simulink model "test_controller"  (R2020a)
settings: Solver=ode1  StartTime=0.0  StopTime=100  FixedStep=0.01  RelTol=1e-3
InitFcn:
  | Initialization;
values from neighbouring files (symbols this model uses):
  ics = JsonLoad('ics.json')    [Initialization.m]
  params = JsonLoad('params.json')    [Initialization.m]
undefined symbols (not defined in the file or in its folder): sim_, U_initial
libraries: sharedtransform x2, dspinverses x2, simulink x2, dspmtrx3 x1, sharedutil x1
(part 1 of 2)
settings Model: NumberOfSteps=100  Creator=arthus  LastModifiedBy=hs293go
settings DataIOCC: ReturnWorkspaceOutputs=off
settings DebuggingCC: ArithmeticOperatorsInVariantConditions=warning
settings SFSimCC: SimUseLocalCustomCode=off  CustomCodeUndefinedFunction=UseInterfaceOnly
settings RTWCC: RTWUseLocalCustomCode=off
settings CodeAppCC: StateflowObjectComments=on

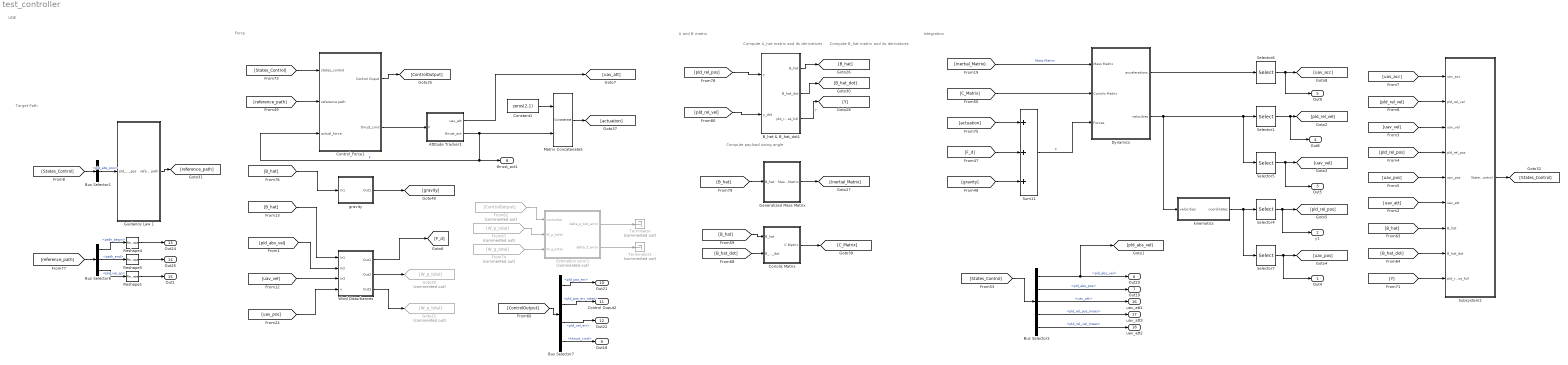
== system test_controller ==
  note: Compute B_hat matrix and its derivatives
  note: Force
  note: A and B matrix
  note: Target Path
  note: Compute A_hat matrix and its derivatives
  note: Integration
  note: Compute payload swing angle
  note: UDE
  Attitude Tracker1 : Subsystem
  B_hat & B_hat_dot1 : Subsystem
  Bus Selector1 : BusSelector  OutputSignals=pld_abs_pos
  Bus Selector2 : BusSelector  OutputSignals=pld_abs_vel,pld_abs_pos,uav_att,pld_rel_pos_meas,pld_rel_vel_meas
  Bus Selector6 : BusSelector  OutputSignals=path_begin,path_end,pld_vel_sp
  Bus Selector7 : BusSelector  OutputSignals=pld_pos_err,pld_pos_err_rates,pld_vel_err,thrust_cmd
  Constant1 : Constant  Value=zeros(2,1)
  Control_Force1 : Subsystem
  Coriolis Matrix : Subsystem
  Dynamics : Subsystem
  Estimation error1 : Subsystem  Commented=on
  From62 : From  Commented=on  GotoTag=ControlOutput
  From67 : From  Commented=on  GotoTag=W_p_total
  From74 : From  Commented=on  GotoTag=W_q_total
  Generalized Mass Matrix : Subsystem
  Goto20 : Goto  Commented=on  GotoTag=W_p_total
  Goto22 : Goto  Commented=on  GotoTag=W_q_total
  Guidance Law 1 : Subsystem
  Matrix Concatenate5 : Concatenate  Mode=Multidimensional array
  Reshape1 : Reshape  OutputDimensionality=Column vector (2-D)
  Reshape4 : Reshape  OutputDimensionality=Column vector (2-D)
  Reshape5 : Reshape  OutputDimensionality=Column vector (2-D)
  Selector1 : Selector  InputPortWidth=5  IndexOptions=Index vector (dialog)  Indices=[1 2]  OutputSizes=1
  Selector4 : Selector  InputPortWidth=5  IndexOptions=Index vector (dialog)  Indices=[1 2]  OutputSizes=1
  Selector5 : Selector  InputPortWidth=5  IndexOptions=Index vector (dialog)  Indices=[3 4 5]  OutputSizes=1
  Selector6 : Selector  InputPortWidth=5  IndexOptions=Index vector (dialog)  Indices=[3 4 5]  OutputSizes=1
  Selector7 : Selector  InputPortWidth=5  IndexOptions=Index vector (dialog)  Indices=[3 4 5]  OutputSizes=1
  Subsystem2 : Subsystem
  Sum11 : Sum  Inputs=+++
  Terminator : Terminator  Commented=on
  Terminator2 : Terminator  Commented=on
  Wind Disturbances : Subsystem
  gravity : Subsystem
  kinematics : Subsystem
  Out4 : Outport  SignalName=uav_pos
  y1 : Outport  Port=2  SignalName=pld_rel_pos
  Out5 : Outport  Port=3  SignalName=uav_vel
  Out8 : Outport  Port=4  SignalName=pld_rel_vel
  Out9 : Outport  Port=5  SignalName=uav_acc
  Out20 : Outport  Port=6  SignalName=pld_abs_vel
  Out19 : Outport  Port=7  SignalName=pld_abs_pos
  thrust_act1 : Outport  Port=8  SignalName=thrust_act  VectorParamsAs1DForOutWhenUnconnected=off
  Out18 : Outport  Port=9  SignalName=thrust_cmd
  Out21 : Outport  Port=10  SignalName=pld_pos_err
  Control Ouput2 : Outport  Port=11  SignalName=pld_pos_err_rates
  Out22 : Outport  Port=12  SignalName=pld_vel_err
  Out24 : Outport  Port=13  SignalName=path_begin
  Out25 : Outport  Port=14  SignalName=path_end
  Out1 : Outport  Port=15  SignalName=pld_vel_sp
  uav_att1 : Outport  Port=16  SignalName=uav_att  VectorParamsAs1DForOutWhenUnconnected=off
  uav_att3 : Outport  Port=17  SignalName=pld_rel_pos_meas  VectorParamsAs1DForOutWhenUnconnected=off
  uav_att2 : Outport  Port=18  SignalName=pld_rel_vel_meas  VectorParamsAs1DForOutWhenUnconnected=off
  wires:
  Control_Force1/1(Control Ouput) -> [ControlOutput]
  Reshape5/1 -> Out25/1
  Constant1/1 -> Matrix Concatenate5/1
  Subsystem2/1(States_Control) -> [States_Control]
  B_hat & B_hat_dot1/2(B_hat_dot) -> [B_hat_dot]
  [B_hat] -> gravity/1(In1)
  Bus Selector6/1 -> Reshape4/1  "<path_begin>"
  Selector5/1 -> [uav_vel], Out5/1
  [Inertial_Matrix] -> Dynamics/1(Mass Matrix)  "Mass Matrix"
  Attitude Tracker1/2(thrust_act) -> Control_Force1/3(actual_force), thrust_act1/1, Matrix Concatenate5/2  "F"
  [reference_path] -> Control_Force1/2(reference path)
  [gravity] -> Sum11/3
  [B_hat] -> Generalized Mass Matrix/1(B_hat)
  Selector7/1 -> [uav_pos], Out4/1
  Bus Selector7/3 -> Out22/1  "<pld_vel_err>"
  Bus Selector2/1 -> [pld_abs_vel], Out20/1  "<pld_abs_vel>"
  From67/1 -> Estimation error1/2(W_p_total)
  Coriolis Matrix/1(C Matrix) -> [C_Matrix]
  Bus Selector2/2 -> Out19/1  "<pld_abs_pos>"
  Dynamics/2(velocities) -> kinematics/1(velocities), Selector5/1, Selector1/1
  [F_d] -> Sum11/2
  [B_hat] -> Subsystem2/7(B_hat)
  Generalized Mass Matrix/1(Mass Matrix) -> [Inertial_Matrix]
  [B_hat_dot] -> Subsystem2/8(B_hat_dot)
  Selector6/1 -> [uav_acc], Out9/1
  Bus Selector6/2 -> Reshape5/1  "<path_end>"
  Sum11/1 -> Dynamics/3(Forces)  "F"
  [Y] -> Subsystem2/9(pld_rel_pos_full)
  Control_Force1/2(thrust_cmd) -> Attitude Tracker1/1(F)
  Selector1/1 -> Out8/1, [pld_rel_vel]
  Matrix Concatenate5/1 -> [actuation]
  [actuation] -> Sum11/1
  B_hat & B_hat_dot1/3(pld_rel_pos_full) -> [Y]  "Y"
  [States_Control] -> Bus Selector2/1
  [ControlOutput] -> Bus Selector7/1
  [pld_rel_pos] -> B_hat & B_hat_dot1/1(y)
  Bus Selector7/2 -> Control Ouput2/1  "<pld_pos_err_rates>"
  [reference_path] -> Bus Selector6/1
  Guidance Law 1/1(reference path) -> [reference_path]
  [States_Control] -> Control_Force1/1(states_control)
  [C_Matrix] -> Dynamics/2(Coriolis Matrix)
  Selector4/1 -> [pld_rel_pos], y1/1
  kinematics/1(coordinates) -> Selector7/1, Selector4/1
  B_hat & B_hat_dot1/1(B_hat) -> [B_hat]
  [pld_rel_vel] -> B_hat & B_hat_dot1/2(y_dot)
  Dynamics/1(accelerations) -> Selector6/1
  Bus Selector7/1 -> Out21/1  "<pld_pos_err>"
  [B_hat] -> Coriolis Matrix/1(B_hat)
  Reshape4/1 -> Out24/1
  [B_hat_dot] -> Coriolis Matrix/2(B_hat_dot)
  Attitude Tracker1/1(uav_att) -> [uav_att]
  gravity/1(Out1) -> [gravity]
  From62/1 -> Estimation error1/1(controller)
  From74/1 -> Estimation error1/3(W_q_total)
  [B_hat] -> Wind Disturbances/1(In1)
  [uav_vel] -> Wind Disturbances/3(In3)
  [uav_pos] -> Wind Disturbances/4(x)
  Wind Disturbances/1(Out1) -> [F_d]
  Wind Disturbances/2(Out2) -> Goto20/1
  Wind Disturbances/3(Out3) -> Goto22/1
  Estimation error1/1(delta_p_bot_error) -> Terminator/1
  Estimation error1/2(delta_T_error) -> Terminator2/1
  [uav_att] -> Subsystem2/6(uav_att)
  Bus Selector2/3 -> uav_att1/1  "<uav_att>"
  [uav_vel] -> Subsystem2/3(uav_vel)
  [pld_rel_pos] -> Subsystem2/4(pld_rel_pos)
  [uav_pos] -> Subsystem2/5(uav_pos)
  [pld_rel_vel] -> Subsystem2/2(pld_rel_vel)
  [uav_acc] -> Subsystem2/1(uav_acc)
  [pld_abs_vel] -> Wind Disturbances/2(In2)
  Bus Selector2/5 -> uav_att2/1  "<pld_rel_vel_meas>"
  Bus Selector2/4 -> uav_att3/1  "<pld_rel_pos_meas>"
  Bus Selector7/4 -> Out18/1  "<thrust_cmd>"
  [States_Control] -> Bus Selector1/1
  Bus Selector1/1 -> Guidance Law 1/1(pld_abs_pos)  "<pld_abs_pos>"
  Reshape1/1 -> Out1/1
  Bus Selector6/3 -> Reshape1/1  "<pld_vel_sp>"

== system test_controller/Attitude Tracker1 ==
  F : Inport
  Attitude Dynamics : Subsystem
  Attitude Tracker : Subsystem
  Atttitude Extraction : Subsystem
  Constant : Constant  Value=[0 0 1]'  VectorParams1D=off
  Divide : Product  Inputs=*/
  Dot Product : DotProduct  InputSameDT=on  OutDataTypeStr=Inherit: Inherit via internal rule
  Product : Product  Multiplication=Matrix(*)
  Product1 : Product
  Sqrt : Sqrt  SaturateOnIntegerOverflow=on
  Terminator : Terminator
  Terminator1 : Terminator
  uav_att : Outport
  thrust_act : Outport  Port=2  VectorParamsAs1DForOutWhenUnconnected=off
  wires:
  F/1 -> Dot Product/2, Dot Product/1, Divide/1
  Constant/1 -> Product/2
  Product/1 -> Product1/2  "n_z"
  Product1/1 -> thrust_act/1
  Sqrt/1 -> Product1/1, Divide/2
  Dot Product/1 -> Sqrt/1
  Atttitude Extraction/1(R_d) -> Attitude Tracker/1(R_d)
  Atttitude Extraction/2(omega_d) -> Attitude Tracker/2(omega_d)
  Atttitude Extraction/3(omega_d_dot) -> Attitude Tracker/3(omega_d_dot)
  Divide/1 -> Atttitude Extraction/1(n_d)  "n1"
  Attitude Dynamics/4(omega_b) -> Attitude Tracker/5(omega)
  Attitude Dynamics/3(Euler) -> Terminator1/1  "Euler"
  Attitude Dynamics/2(RBI) -> Terminator/1
  Attitude Tracker/1(Torque_in_body_frame) -> Attitude Dynamics/1(MB)  "Mq_b"
  Attitude Dynamics/1(RIB) -> uav_att/1, Attitude Tracker/4(R), Product/1  "IRB"

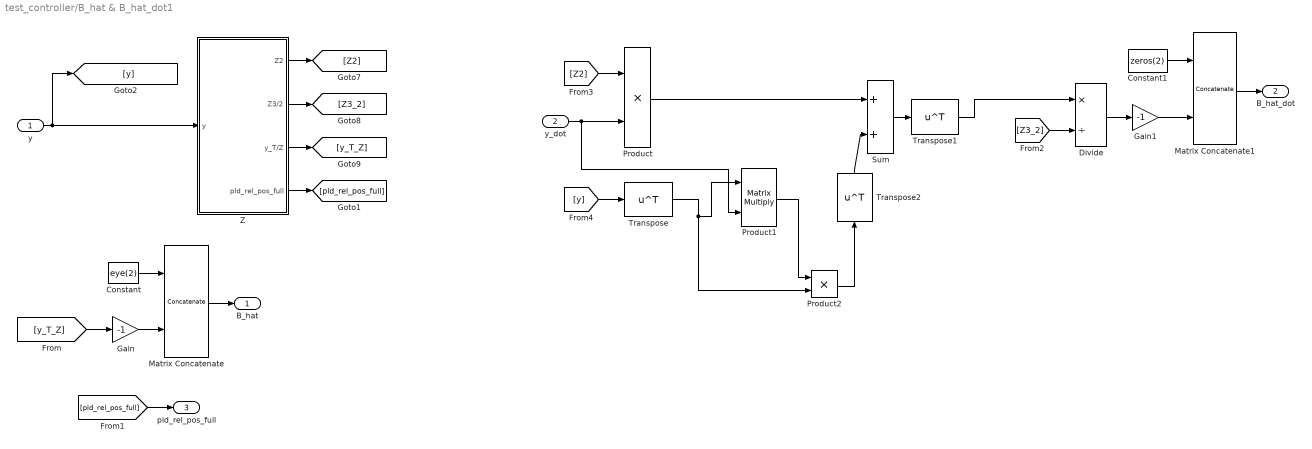
== system test_controller/B_hat & B_hat_dot1 ==
  y : Inport
  y_dot : Inport  Port=2
  Constant : Constant  Value=eye(2)
  Constant1 : Constant  Value=zeros(2)
  Divide : Product  Inputs=*/
  Gain : Gain  Gain=-1
  Gain1 : Gain  Gain=-1
  Matrix Concatenate : Concatenate  Mode=Multidimensional array
  Matrix Concatenate1 : Concatenate  Mode=Multidimensional array
  Product : Product  RndMeth=Zero
  Product1 : Product  Multiplication=Matrix(*)  RndMeth=Zero
  Product2 : Product  RndMeth=Zero
  Sum : Sum
  Transpose : Math  Operator=transpose  SignedPower=on  SaturateOnIntegerOverflow=on
  Transpose1 : Math  Operator=transpose  SignedPower=on  SaturateOnIntegerOverflow=on
  Transpose2 : Math  Operator=transpose  SignedPower=on  SaturateOnIntegerOverflow=on
  Z : Subsystem
  B_hat : Outport  VectorParamsAs1DForOutWhenUnconnected=off
  B_hat_dot : Outport  Port=2  VectorParamsAs1DForOutWhenUnconnected=off
  pld_rel_pos_full : Outport  Port=3  VectorParamsAs1DForOutWhenUnconnected=off
  wires:
  y_dot/1 -> Product/2, Product1/2
  y/1 -> Z/1(y), [y]
  Matrix Concatenate/1 -> B_hat/1
  Matrix Concatenate1/1 -> B_hat_dot/1
  Z/1(Z2) -> [Z2]
  Z/2(Z3/2) -> [Z3_2]
  Z/3(y_T/Z) -> [y_T_Z]
  [y_T_Z] -> Gain/1
  Constant/1 -> Matrix Concatenate/1
  Gain/1 -> Matrix Concatenate/2
  Z/4(pld_rel_pos_full) -> [pld_rel_pos_full]
  [pld_rel_pos_full] -> pld_rel_pos_full/1
  Constant1/1 -> Matrix Concatenate1/1
  [Z3_2] -> Divide/2
  Sum/1 -> Transpose1/1
  [Z2] -> Product/1
  [y] -> Transpose/1
  Transpose/1 -> Product1/1, Product2/2
  Product1/1 -> Product2/1
  Divide/1 -> Gain1/1
  Gain1/1 -> Matrix Concatenate1/2
  Product2/1 -> Transpose2/1
  Product/1 -> Sum/1
  Transpose1/1 -> Divide/1
  Transpose2/1 -> Sum/2

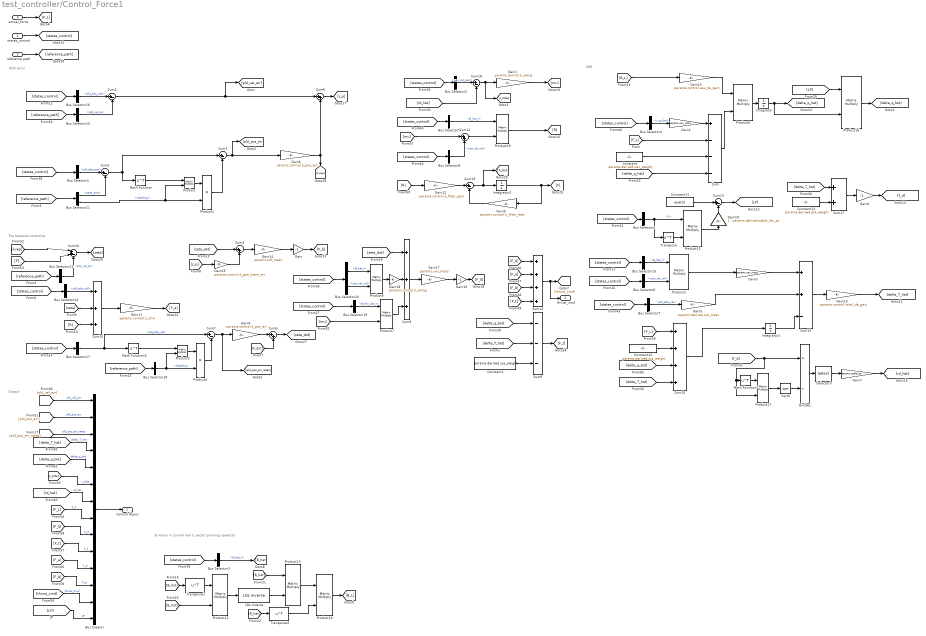
== system test_controller/Control_Force1 ==
  note: Output
  note: Path error
  note: The baseline controller
  note: B matrix in control law (L vector pointing upwards)
  note: UDE
  states_control : Inport
  reference path : Inport  Port=2
  actual_force : Inport  Port=3
  Bus Creator : BusCreator  Inputs=14
  Bus Selector1 : BusSelector  OutputSignals=pld_abs_pos
  Bus Selector10 : BusSelector  OutputSignals=pld_vel_sp
  Bus Selector11 : BusSelector  OutputSignals=path_end,heading
  Bus Selector13 : BusSelector  OutputSignals=pld_vel_sp
  Bus Selector{7,14,16..17} (4 alike) : BusSelector  OutputSignals=pld_abs_vel
  Bus Selector15 : BusSelector  OutputSignals=B_hat_l
  Bus Selector18 : BusSelector  OutputSignals=heading
  Bus Selector19 : BusSelector  OutputSignals=B_hat_dot_l
  Bus Selector2 : BusSelector  OutputSignals=uav_rel_pos
  Bus Selector20 : BusSelector  OutputSignals=B_hat_l,uav_rel_vel
  Bus Selector3 : BusSelector  OutputSignals=B_hat_l
  Bus Selector4 : BusSelector  OutputSignals=v_q_dot
  Bus Selector5 : BusSelector  OutputSignals=L
  Bus Selector6 : BusSelector  OutputSignals=uav_rel_vel
  Bus Selector8 : BusSelector  OutputSignals=uav_rel_vel
  Bus Selector9 : BusSelector  OutputSignals=B_hat_l
  Constant : Constant  Value=params.derived.uav_weight
  Constant1 : Constant  Value=params.derived.sys_weight
  Constant11 : Constant  Value=eye(3)
  Constant12 : Constant  Value=params.derived.sys_weight
  Constant13 : Constant  Value=params.derived.pld_weight
  Divide1 : Product  Inputs=*/
  Gain : Gain  Gain=-1
  Gain1 : Gain  Gain=params.control.k_swing
  Gain10 : Gain  Gain=params.control.uav_de_gain
  Gain11 : Gain  Gain=-params.control.k_trim
  Gain12 : Gain  Gain=params.control.k_filter_gain
  Gain13 : Gain  Gain=params.control.total_de_gain
  Gain14 : Gain  Gain=params.pld_mass
  Gain15 : Gain  Gain=params.control.k_gen_trans_err
  Gain16 : Gain  Gain=-1
  Gain17 : Gain  Gain=params.uav_mass
  Gain18 : Gain  Gain=params.control.k_swing
  Gain19 : Gain  Gain=1 / params.derived.cable_len_sq
  Gain2 : Gain  Gain=params.uav_mass
  Gain3 : Gain  Gain=params.uav_mass
  Gain4 : Gain  Gain=params.control.k_pos_err
  Gain5 : Gain  Gain=params.derived.sys_mass
  Gain6 : Gain  Gain=-1
  Gain7 : Gain  Gain=params.cable_len
  Gain8 : Gain  Gain=params.control.k_pos_err
  Gain9 : Gain  Gain=params.control.k_filter_leak
  Integrator : Integrator
  Integrator1 : Integrator
  Integrator2 : Integrator
  LDL Inverse : dspinverses/LDL Inverse  errmode=Error
      settings: SourceProductBaseCode=DS
  Math Function : Math  Operator=transpose  SignedPower=on  SaturateOnIntegerOverflow=on
  Math Function3 : Math  Operator=transpose  SignedPower=on  SaturateOnIntegerOverflow=on
  Math Function4 : Math  Operator=transpose  SignedPower=on  SaturateOnIntegerOverflow=on
  Product{,2..3,7..9,12..17,19} (13 alike) : Product  Multiplication=Matrix(*)
  Product1 : Product
  Product4 : Product
  Selector3 : Selector  InputPortWidth=3  IndexOptions=Index vector (dialog)  Indices=[1 2]  OutputSizes=1
  Sqrt6 : Sqrt  SaturateOnIntegerOverflow=on
  Sum : Sum  Inputs=+---
  Sum{1..3,7,13,18..19} (7 alike) : Sum  Inputs=|+-
  Sum10 : Sum  Inputs=+++
  Sum{4..6,12} (4 alike) : Sum  Inputs=|++
  Sum14 : Sum  Inputs=++++
  Sum15 : Sum  Inputs=++-
  Sum16 : Sum  Inputs=++++
  Sum17 : Sum
  Sum20 : Sum  Inputs=|++-
  Sum8 : Sum  Inputs=+++
  Sum9 : Sum  Inputs=---
  Transpose : Math  Operator=transpose  SignedPower=on  SaturateOnIntegerOverflow=on
  Transpose1 : Math  Operator=transpose  SignedPower=on  SaturateOnIntegerOverflow=on
  Transpose3 : Math  Operator=transpose  SignedPower=on  SaturateOnIntegerOverflow=on
  Control Ouput : Outport  VectorParamsAs1DForOutWhenUnconnected=off
  thrust_cmd : Outport  Port=2  VectorParamsAs1DForOutWhenUnconnected=off
  wires:
  Sum3/1 -> Gain4/1, [pld_pos_err]
  Sum1/1 -> Sum3/1, Math Function/1
  Math Function/1 -> Product/1
  Product/1 -> Product1/1
  Product1/1 -> Sum3/2
  Bus Selector6/1 -> Product2/2  "<uav_rel_vel>"
  Bus Selector7/1 -> Gain5/1  "<pld_abs_vel>"
  Sum2/1 -> Sum6/1, [pld_vel_err]
  Sum14/1 -> thrust_cmd/1, [thrust_cmd]
  [B_hat] -> Transpose1/1
  Transpose1/1 -> Product12/1
  [B_hat] -> Product12/2
  Product12/1 -> LDL Inverse/1
  LDL Inverse/1 -> Product13/2
  [B_hat] -> Product13/1
  Transpose3/1 -> Product14/2
  [B_hat] -> Transpose3/1
  Product13/1 -> Product14/1
  Product14/1 -> [B_L]
  [B_L] -> Gain10/1
  Gain10/1 -> Product8/1
  Integrator/1 -> Product16/2, [delta_q_hat]
  [delta_q_hat] -> Sum/4
  Constant/1 -> Sum/3
  [F_L] -> Sum/2
  Gain2/1 -> Sum/1
  Sum/1 -> Product8/2
  Product8/1 -> Integrator/1
  Constant11/1 -> Sum13/1
  Product15/1 -> Gain19/1
  Sum13/1 -> [LP]
  [LP] -> Product16/1
  Product16/1 -> [delta_q_bot]
  Bus Selector15/1 -> Product2/1  "<B_hat_l>"
  Product2/1 -> Gain3/1
  Gain3/1 -> Sum15/1
  Gain5/1 -> Sum15/2
  Sum15/1 -> Gain13/1
  Integrator1/1 -> Sum15/3
  [F_L] -> Sum16/1
  Constant12/1 -> Sum16/2
  [delta_q_bot] -> Sum16/3
  [delta_T_hat] -> Sum16/4
  [delta_T_hat] -> Sum17/1
  Constant13/1 -> Sum17/2
  Sum17/1 -> Gain6/1
  Gain6/1 -> [f_d]
  Selector3/1 -> Gain7/1
  Gain7/1 -> [rd_hat]
  Product17/1 -> Sqrt6/1
  [f_d] -> Product17/2, Math Function4/1, Divide1/1
  Divide1/1 -> Selector3/1
  Sqrt6/1 -> Divide1/2
  Math Function4/1 -> Product17/1
  Sum6/1 -> [s_p]
  Bus Selector16/1 -> Sum2/1  "<pld_abs_vel>"
  Sum18/1 -> [r_tilde], Gain1/1
  Gain1/1 -> [mu]
  states_control/1 -> [states_control]
  [states_control] -> Bus Selector1/1
  Bus Selector1/1 -> Sum1/1  "<pld_abs_pos>"
  [states_control] -> Bus Selector2/1
  Bus Selector2/1 -> Sum18/1  "<uav_rel_pos>"
  [states_control] -> Bus Selector3/1
  Bus Selector3/1 -> [B_hat]  "<B_hat_l>"
  [states_control] -> Bus Selector4/1
  Bus Selector4/1 -> Gain2/1  "<v_q_dot>"
  [states_control] -> Bus Selector5/1
  Bus Selector5/1 -> Product15/1, Transpose/1  "<L>"
  [states_control] -> Bus Selector6/1
  [states_control] -> Bus Selector7/1
  [mu] -> Sum12/1
  Bus Selector8/1 -> Sum12/2  "<uav_rel_vel>"
  [states_control] -> Bus Selector8/1
  Sum12/1 -> Product19/2
  Bus Selector9/1 -> Product19/1  "<B_hat_l>"
  [states_control] -> Bus Selector9/1
  Product19/1 -> [R]
  [F_0] -> Sum14/1
  [F_a] -> Sum14/2
  [F_b] -> Sum14/3
  [F_t] -> Sum14/4
  Integrator2/1 -> Gain9/1, [F]
  Sum19/1 -> [F_dot], Integrator2/1
  Gain9/1 -> Sum19/2
  [R] -> Gain12/1
  Gain12/1 -> Sum19/1
  Sum20/1 -> [zeta]
  Gain4/1 -> [kvep], Sum6/2
  [kvep] -> Sum20/1
  [F] -> Sum20/2
  reference path/1 -> [reference_path]
  [reference_path] -> Bus Selector10/1
  Bus Selector10/1 -> Sum2/2  "<pld_vel_sp>"
  Bus Selector11/1 -> Sum1/2  "<path_end>"
  [reference_path] -> Bus Selector11/1
  Bus Selector11/2 -> Product1/2, Product/2  "<heading>"
  [reference_path] -> Bus Selector13/1
  Bus Selector13/1 -> Sum20/3  "<pld_vel_sp>"
  Sum4/1 -> Gain14/1
  Gain16/1 -> [F_0]
  Gain11/1 -> [F_a]
  Sum9/1 -> [F_t]
  Sum10/1 -> Gain11/1
  Constant1/1 -> Sum9/3
  [states_control] -> Bus Selector14/1
  Bus Selector14/1 -> Sum10/1  "<pld_abs_vel>"
  [zeta] -> Sum10/2
  [R] -> Sum10/3
  Sum16/1 -> Integrator1/1
  [delta_q_bot] -> Sum9/1
  [rd_hat] -> Sum18/2
  Gain13/1 -> [delta_T_hat]
  [states_control] -> Bus Selector15/1
  [delta_T_hat] -> Sum9/2
  [states_control] -> Bus Selector16/1
  Gain/1 -> [F_b]
  [F_dot] -> Sum5/2
  Sum5/1 -> [zeta_dot]
  [zeta_dot] -> Sum4/1
  Gain14/1 -> Gain/1
  Gain15/1 -> Sum4/2
  [s_p] -> Gain15/1
  Gain8/1 -> Sum5/1
  [states_control] -> Bus Selector17/1
  Bus Selector17/1 -> Sum7/1, Math Function3/1  "<pld_abs_vel>"
  [reference_path] -> Bus Selector18/1
  Bus Selector18/1 -> Product3/2, Product4/2  "<heading>"
  Product3/1 -> Product4/1
  Math Function3/1 -> Product3/1
  Product4/1 -> Sum7/2
  Sum7/1 -> [pld_pos_err_rates], Gain8/1
  Gain17/1 -> Gain16/1
  Sum8/1 -> Gain17/1
  [zeta_dot] -> Sum8/1
  Gain18/1 -> Sum8/2
  [states_control] -> Bus Selector19/1
  Bus Selector19/1 -> Product7/1  "<B_hat_dot_l>"
  Product7/1 -> Sum8/3
  [mu] -> Product7/2
  Product9/1 -> Gain18/1
  Bus Selector20/1 -> Product9/1  "<B_hat_l>"
  [states_control] -> Bus Selector20/1
  Bus Selector20/2 -> Product9/2  "<uav_rel_vel>"
  Bus Creator/1 -> Control Ouput/1
  [pld_vel_err] -> Bus Creator/1  "pld_vel_err"
  [pld_pos_err] -> Bus Creator/2  "pld_pos_err"
  [delta_T_hat] -> Bus Creator/4  "delta_T_hat"
  [delta_q_bot] -> Bus Creator/5  "delta_q_bot"
  [r_tilde] -> Bus Creator/6  "r_tilde"
  [rd_hat] -> Bus Creator/7  "rd_hat"
  [F_L] -> Bus Creator/8  "F_L"
  [F_0] -> Bus Creator/9  "F_0"
  [F_t] -> Bus Creator/10  "F_t"
  [F_a] -> Bus Creator/11  "F_a"
  [F_b] -> Bus Creator/12  "F_b"
  [thrust_cmd] -> Bus Creator/13  "thrust_cmd"
  [LP] -> Bus Creator/14  "LP"
  Gain19/1 -> Sum13/2
  Transpose/1 -> Product15/2
  actual_force/1 -> [F_L]
  [pld_pos_err_rates] -> Bus Creator/3  "pld_pos_err_rates"

== system test_controller/Coriolis Matrix ==
  B_hat : Inport
  B_hat_dot : Inport  Port=2
  Constant : Constant  Value=[zeros(2,3);zeros(3)]  VectorParams1D=off
  Gain4 : Gain  Gain=params.pld_mass
  Gain5 : Gain  Gain=params.pld_mass
  Matrix Concatenate : Concatenate  Mode=Multidimensional array  ConcatenateDimension=2
  Matrix Concatenate1 : Concatenate  Mode=Multidimensional array
  Product1 : Product  Multiplication=Matrix(*)
  Transpose3 : Math  Operator=transpose  SignedPower=on  SaturateOnIntegerOverflow=on
  C Matrix : Outport  VectorParamsAs1DForOutWhenUnconnected=off
  wires:
  B_hat_dot/1 -> Gain4/1, Product1/2
  Matrix Concatenate1/1 -> Matrix Concatenate/1
  Constant/1 -> Matrix Concatenate/2
  B_hat/1 -> Transpose3/1
  Transpose3/1 -> [B_hatT]
  Gain5/1 -> Matrix Concatenate1/1
  [B_hatT] -> Product1/1
  Matrix Concatenate/1 -> C Matrix/1
  Product1/1 -> Gain5/1
  Gain4/1 -> Matrix Concatenate1/2

== system test_controller/Dynamics ==
  Mass Matrix : Inport
  Coriolis Matrix : Inport  Port=2
  Forces : Inport  Port=3
  Constant8 : Constant  Value=[ics.pld_rel_vel; ics.uav_vel]  VectorParams1D=off
  Integrator2 : Integrator  InitialConditionSource=external  InitialCondition=U_initial
  LDL Inverse : dspinverses/LDL Inverse  errmode=Error
      settings: SourceProductBaseCode=DS
  Product2 : Product  Multiplication=Matrix(*)  RndMeth=Zero
  Product6 : Product  Multiplication=Matrix(*)
  Sum7 : Sum  Inputs=+-
  accelerations : Outport
  velocities : Outport  Port=2
  wires:
  Integrator2/1 -> Product6/2, velocities/1
  Sum7/1 -> Product2/2  "F"
  Constant8/1 -> Integrator2/2
  Forces/1 -> Sum7/1
  LDL Inverse/1 -> Product2/1
  Product6/1 -> Sum7/2
  Coriolis Matrix/1 -> Product6/1
  Product2/1 -> Integrator2/1, accelerations/1  "u_dot"
  Mass Matrix/1 -> LDL Inverse/1

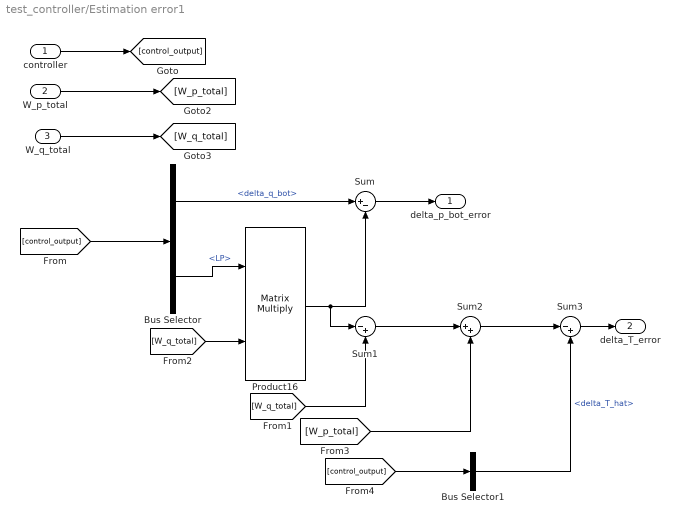
== system test_controller/Estimation error1 ==
  controller : Inport
  W_p_total : Inport  Port=2
  W_q_total : Inport  Port=3
  Bus Selector : BusSelector  OutputSignals=delta_q_bot,LP
  Bus Selector1 : BusSelector  OutputSignals=delta_T_hat
  Product16 : Product  Multiplication=Matrix(*)
  Sum : Sum  Inputs=|+-
  Sum1 : Sum  Inputs=|-+
  Sum2 : Sum  Inputs=|++
  Sum3 : Sum  Inputs=|-+
  delta_p_bot_error : Outport  VectorParamsAs1DForOutWhenUnconnected=off
  delta_T_error : Outport  Port=2  VectorParamsAs1DForOutWhenUnconnected=off
  wires:
  W_p_total/1 -> [W_p_total]
  Bus Selector1/1 -> Sum3/2  "<delta_T_hat>"
  Product16/1 -> Sum1/1, Sum/2
  [control_output] -> Bus Selector1/1
  [control_output] -> Bus Selector/1
  Sum2/1 -> Sum3/1
  [W_p_total] -> Sum2/2
  [W_q_total] -> Sum1/2
  Sum1/1 -> Sum2/1
  Sum3/1 -> delta_T_error/1
  Sum/1 -> delta_p_bot_error/1
  [W_q_total] -> Product16/2
  Bus Selector/2 -> Product16/1  "<LP>"
  controller/1 -> [control_output]
  Bus Selector/1 -> Sum/1  "<delta_q_bot>"
  W_q_total/1 -> [W_q_total]

== system test_controller/Generalized Mass Matrix ==
  B_hat : Inport
  Constant : Constant  Value=params.derived.sys_mass*eye(3)
  Gain1 : Gain  Gain=params.pld_mass
  Gain2 : Gain  Gain=params.pld_mass
  Gain3 : Gain  Gain=params.pld_mass
  Matrix Concatenate : Concatenate  Mode=Multidimensional array  ConcatenateDimension=2
  Matrix Concatenate1 : Concatenate  Mode=Multidimensional array
  Matrix Concatenate2 : Concatenate  Mode=Multidimensional array
  Product : Product  Multiplication=Matrix(*)
  Transpose3 : Math  Operator=transpose  SignedPower=on  SaturateOnIntegerOverflow=on
  Mass Matrix : Outport  VectorParamsAs1DForOutWhenUnconnected=off
  wires:
  B_hat/1 -> Transpose3/1, [B_hat]
  Matrix Concatenate1/1 -> Matrix Concatenate/1
  Matrix Concatenate2/1 -> Matrix Concatenate/2
  Matrix Concatenate/1 -> Mass Matrix/1
  Product/1 -> Gain1/1
  Transpose3/1 -> [B_hatT]
  [B_hatT] -> Product/1
  Gain1/1 -> Matrix Concatenate1/1
  Gain2/1 -> Matrix Concatenate1/2
  Constant/1 -> Matrix Concatenate2/2
  [B_hat] -> Gain2/1
  Gain3/1 -> Matrix Concatenate2/1
  [B_hat] -> Product/2
  [B_hatT] -> Gain3/1

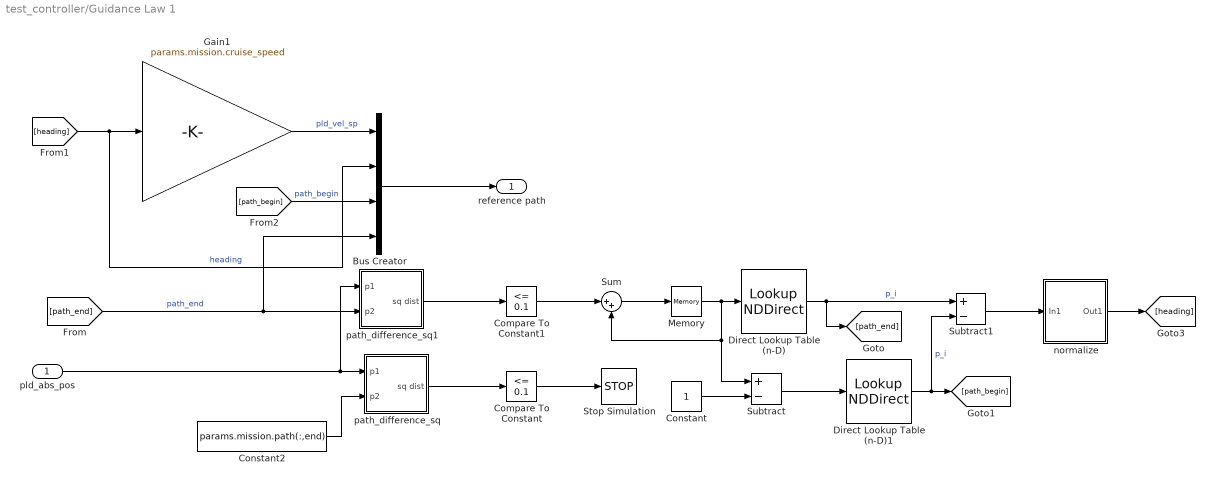
== system test_controller/Guidance Law 1 ==
  pld_abs_pos : Inport
  Bus Creator : BusCreator  Inputs=4
  Compare To Constant : simulink/Logic and Bit Operations/Compare To Constant  relop=<=  const=0.1  OutDataTypeStr=boolean
  Compare To Constant1 : simulink/Logic and Bit Operations/Compare To Constant  relop=<=  const=0.1  OutDataTypeStr=uint8
  Constant : Constant
  Constant2 : Constant  Value=params.mission.path(:,end)
  Direct Lookup Table (n-D) : LookupNDDirect  InputsSelectThisObjectFromTable=Vector  Table=params.mission.path
  Direct Lookup Table (n-D)1 : LookupNDDirect  InputsSelectThisObjectFromTable=Vector  Table=params.mission.path
  Gain1 : Gain  Gain=params.mission.cruise_speed
  Memory : Memory  InitialCondition=1
  Stop Simulation : Stop
  Subtract : Sum  Inputs=+-
  Subtract1 : Sum  Inputs=+-
  Sum : Sum  Inputs=|++
  normalize : Subsystem
  path_difference_sq : Subsystem
  path_difference_sq1 : Subsystem
  reference path : Outport  VectorParamsAs1DForOutWhenUnconnected=off
  wires:
  Direct Lookup Table (n-D)/1 -> [path_end], Subtract1/1  "p_i"
  pld_abs_pos/1 -> path_difference_sq/1(p1), path_difference_sq1/1(p1)
  Bus Creator/1 -> reference path/1
  Compare To Constant/1 -> Stop Simulation/1
  Gain1/1 -> Bus Creator/1  "pld_vel_sp"
  [path_end] -> path_difference_sq1/2(p2), Bus Creator/4  "path_end"
  Memory/1 -> Subtract/1, Sum/2, Direct Lookup Table (n-D)/1
  Constant/1 -> Subtract/2
  Sum/1 -> Memory/1
  [path_begin] -> Bus Creator/3  "path_begin"
  Direct Lookup Table (n-D)1/1 -> [path_begin], Subtract1/2  "p_i"
  normalize/1(Out1) -> [heading]
  Subtract1/1 -> normalize/1(In1)
  Subtract/1 -> Direct Lookup Table (n-D)1/1
  Constant2/1 -> path_difference_sq/2(p2)
  path_difference_sq1/1(sq dist) -> Compare To Constant1/1
  [heading] -> Bus Creator/2, Gain1/1  "heading"
  path_difference_sq/1(sq dist) -> Compare To Constant/1
  Compare To Constant1/1 -> Sum/1

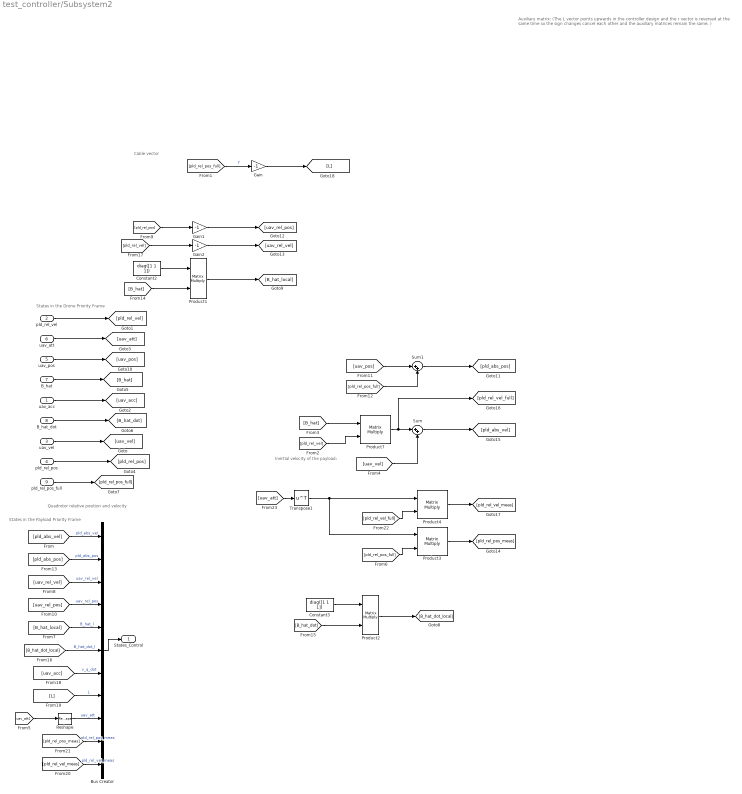
== system test_controller/Subsystem2 ==
  note: Quadrotor relative position and velocity
  note: Auxiliary matrix: (The L vector points upwards in the controller design and the r vector is reversed at the same time so
      | the sign changes cancel each other and the auxiliary matrices remain the same.  )
  note: Cable vector
  note: Inertial velocity of the payload:
  note: States in the Drone Priority Frame
  note: States in the Payload Priority Frame
  uav_acc : Inport
  pld_rel_vel : Inport  Port=2
  uav_vel : Inport  Port=3
  pld_rel_pos : Inport  Port=4
  uav_pos : Inport  Port=5
  uav_att : Inport  Port=6
  B_hat : Inport  Port=7
  B_hat_dot : Inport  Port=8
  pld_rel_pos_full : Inport  Port=9
  Bus Creator : BusCreator  Inputs=11
  Constant2 : Constant  Value=diag([1 1 1])
  Constant3 : Constant  Value=diag([1 1 1])
  Gain : Gain  Gain=-1
  Gain1 : Gain  Gain=-1
  Gain2 : Gain  Gain=-1
  Product{1..4,7} (5 alike) : Product  Multiplication=Matrix(*)
  Reshape : Reshape  OutputDimensionality=Column vector (2-D)
  Sum : Sum  Inputs=|++
  Sum1 : Sum  Inputs=|++
  Transpose1 : Math  Operator=transpose  SaturateOnIntegerOverflow=on
  States_Control : Outport  VectorParamsAs1DForOutWhenUnconnected=off
  wires:
  uav_vel/1 -> [uav_vel]
  uav_acc/1 -> [uav_acc]
  B_hat/1 -> [B_hat]
  pld_rel_pos_full/1 -> [pld_rel_pos_full]
  uav_pos/1 -> [uav_pos]
  Bus Creator/1 -> States_Control/1
  B_hat_dot/1 -> [B_hat_dot]
  [pld_abs_vel] -> Bus Creator/1  "pld_abs_vel"
  [pld_abs_pos] -> Bus Creator/2  "pld_abs_pos"
  [uav_rel_vel] -> Bus Creator/3  "uav_rel_vel"
  [B_hat_dot_local] -> Bus Creator/6  "B_hat_dot_l"
  pld_rel_vel/1 -> [pld_rel_vel]
  uav_att/1 -> [uav_att]
  Gain2/1 -> [uav_rel_vel]
  [pld_rel_pos_full] -> Gain/1  "Y"
  [B_hat_local] -> Bus Creator/5  "B_hat_l"
  [B_hat] -> Product7/1
  [B_hat_dot] -> Product2/2
  [uav_rel_pos] -> Bus Creator/4  "uav_rel_pos"
  Product3/1 -> [pld_rel_pos_meas]
  [pld_rel_pos_full] -> Sum1/2
  Constant2/1 -> Product1/1
  [L] -> Bus Creator/8  "L"
  Constant3/1 -> Product2/1
  [uav_acc] -> Bus Creator/7  "v_q_dot"
  [pld_rel_vel] -> Product7/2
  Transpose1/1 -> Product4/1, Product3/1
  Gain1/1 -> [uav_rel_pos]
  pld_rel_pos/1 -> [pld_rel_pos]
  [uav_att] -> Reshape/1
  [pld_rel_pos] -> Gain1/1
  Product2/1 -> [B_hat_dot_local]
  Sum1/1 -> [pld_abs_pos]
  [uav_pos] -> Sum1/1
  Gain/1 -> [L]
  [pld_rel_pos_meas] -> Bus Creator/10  "pld_rel_pos_meas"
  Product1/1 -> [B_hat_local]
  [pld_rel_pos_full] -> Product3/2
  Sum/1 -> [pld_abs_vel]
  [uav_vel] -> Sum/2
  [pld_rel_vel] -> Gain2/1
  Product7/1 -> [pld_rel_vel_full], Sum/1
  [B_hat] -> Product1/2
  Reshape/1 -> Bus Creator/9  "uav_att"
  [pld_rel_vel_full] -> Product4/2
  [uav_att] -> Transpose1/1
  Product4/1 -> [pld_rel_vel_meas]
  [pld_rel_vel_meas] -> Bus Creator/11  "pld_rel_vel_meas"

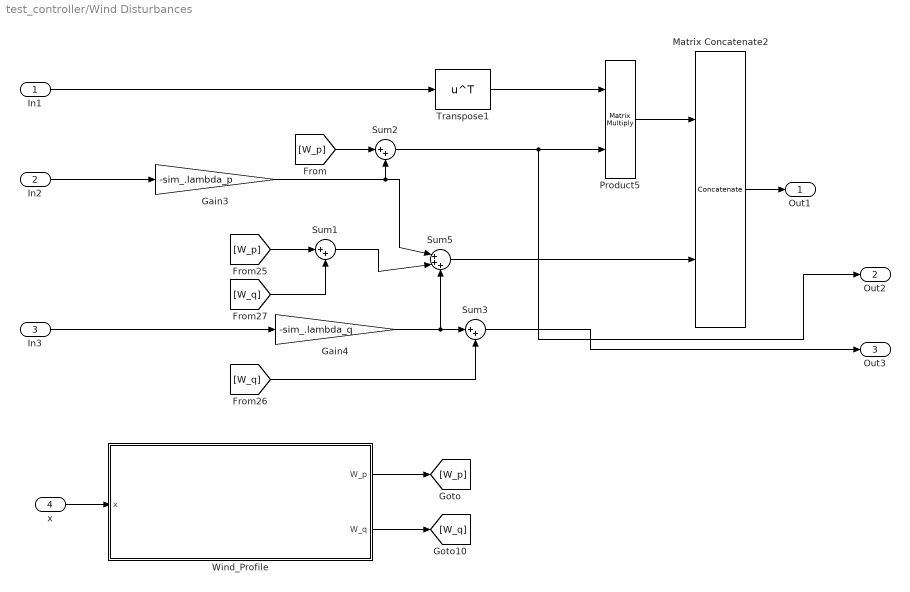
== system test_controller/Wind Disturbances ==
  In1 : Inport
  In2 : Inport  Port=2
  In3 : Inport  Port=3
  x : Inport  Port=4
  Gain3 : Gain  Gain=-sim_.lambda_p
  Gain4 : Gain  Gain=-sim_.lambda_q
  Matrix Concatenate2 : Concatenate  Mode=Multidimensional array
  Product5 : Product  Multiplication=Matrix(*)
  Sum1 : Sum  Inputs=|++
  Sum2 : Sum  Inputs=|++
  Sum3 : Sum  Inputs=|++
  Sum5 : Sum  Inputs=|+++
  Transpose1 : Math  Operator=transpose  SignedPower=on  SaturateOnIntegerOverflow=on
  Wind_Profile : Subsystem
  Out1 : Outport
  Out2 : Outport  Port=2
  Out3 : Outport  Port=3
  wires:
  In1/1 -> Transpose1/1
  Wind_Profile/1(W_p) -> [W_p]
  Transpose1/1 -> Product5/1
  [W_q] -> Sum1/2
  In3/1 -> Gain4/1
  x/1 -> Wind_Profile/1(x)
  Gain3/1 -> Sum2/2, Sum5/1
  Product5/1 -> Matrix Concatenate2/1
  [W_q] -> Sum3/2
  In2/1 -> Gain3/1
  Sum2/1 -> Out2/1, Product5/2
  Sum3/1 -> Out3/1
  [W_p] -> Sum1/1
  Gain4/1 -> Sum3/1, Sum5/3
  Sum5/1 -> Matrix Concatenate2/2
  Wind_Profile/2(W_q) -> [W_q]
  Matrix Concatenate2/1 -> Out1/1
  [W_p] -> Sum2/1
  Sum1/1 -> Sum5/2

== system test_controller/gravity ==
  In1 : Inport
  Constant6 : Constant  Value=sim_.grav  VectorParams1D=off
  Gain2 : Gain  Gain=params.derived.sys_mass
  Gain5 : Gain  Gain=params.pld_mass
  Matrix Concatenate1 : Concatenate  Mode=Multidimensional array
  Product3 : Product  Multiplication=Matrix(*)
  Transpose3 : Math  Operator=transpose  SignedPower=on  SaturateOnIntegerOverflow=on
  Out1 : Outport
  wires:
  Transpose3/1 -> Gain5/1
  Gain5/1 -> Product3/1
  In1/1 -> Transpose3/1
  Product3/1 -> Matrix Concatenate1/1
  Gain2/1 -> Matrix Concatenate1/2
  Matrix Concatenate1/1 -> Out1/1
  Constant6/1 -> Gain2/1, Product3/2

== system test_controller/kinematics ==
  velocities : Inport
  Integrator3 : Integrator  InitialConditionSource=external
  inital position : Constant  Value=[ics.pld_rel_pos; ics.uav_pos]
  coordinates : Outport
  wires:
  inital position/1 -> Integrator3/2
  velocities/1 -> Integrator3/1
  Integrator3/1 -> coordinates/1

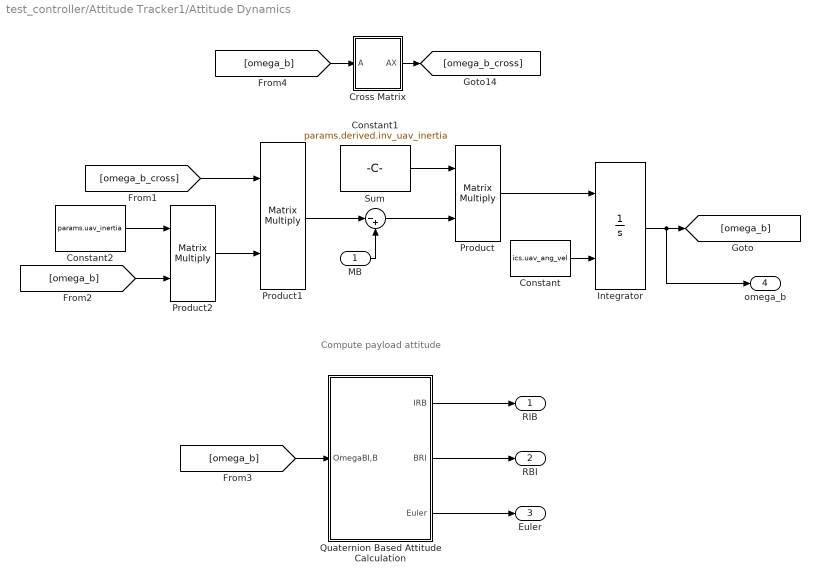
== system test_controller/Attitude Tracker1/Attitude Dynamics ==
  note: Compute payload attitude
  MB : Inport
  Constant : Constant  Value=ics.uav_ang_vel  VectorParams1D=off
  Constant1 : Constant  Value=params.derived.inv_uav_inertia  VectorParams1D=off
  Constant2 : Constant  Value=params.uav_inertia  VectorParams1D=off
  Cross Matrix : Subsystem
  Integrator : Integrator  InitialConditionSource=external
  Product : Product  Multiplication=Matrix(*)
  Product1 : Product  Multiplication=Matrix(*)
  Product2 : Product  Multiplication=Matrix(*)
  Quaternion Based Attitude Calculation : Subsystem
  Sum : Sum  Inputs=|-+
  RIB : Outport  VectorParamsAs1DForOutWhenUnconnected=off
  RBI : Outport  Port=2  VectorParamsAs1DForOutWhenUnconnected=off
  Euler : Outport  Port=3  VectorParamsAs1DForOutWhenUnconnected=off
  omega_b : Outport  Port=4  VectorParamsAs1DForOutWhenUnconnected=off
  wires:
  [omega_b] -> Cross Matrix/1(A)
  Cross Matrix/1(AX) -> [omega_b_cross]
  [omega_b] -> Quaternion Based Attitude Calculation/1(OmegaBI,B)
  Quaternion Based Attitude Calculation/1(IRB) -> RIB/1
  Quaternion Based Attitude Calculation/2(BRI) -> RBI/1
  Quaternion Based Attitude Calculation/3(Euler) -> Euler/1
  Integrator/1 -> omega_b/1, [omega_b]
  Constant/1 -> Integrator/2
  Product/1 -> Integrator/1
  Constant1/1 -> Product/1
  Sum/1 -> Product/2
  MB/1 -> Sum/2
  [omega_b_cross] -> Product1/1
  Product2/1 -> Product1/2
  Constant2/1 -> Product2/1
  [omega_b] -> Product2/2
  Product1/1 -> Sum/1

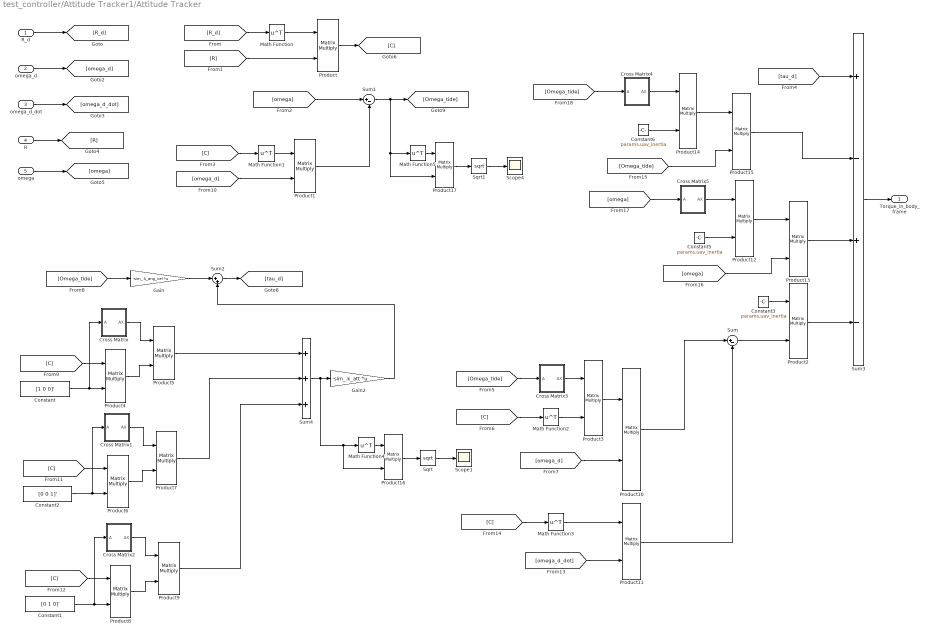
== system test_controller/Attitude Tracker1/Attitude Tracker ==
  R_d : Inport
  omega_d : Inport  Port=2
  omega_d_dot : Inport  Port=3
  R : Inport  Port=4
  omega : Inport  Port=5
  Constant : Constant  Value=[1 0 0]'
  Constant1 : Constant  Value=[0 1 0]'
  Constant2 : Constant  Value=[0 0 1]'
  Constant3 : Constant  Value=params.uav_inertia  VectorParams1D=off
  Constant5 : Constant  Value=params.uav_inertia  VectorParams1D=off
  Constant6 : Constant  Value=params.uav_inertia  VectorParams1D=off
  Cross Matrix : Subsystem
  Cross Matrix1 : Subsystem
  Cross Matrix2 : Subsystem
  Cross Matrix3 : Subsystem
  Cross Matrix4 : Subsystem
  Cross Matrix5 : Subsystem
  Gain : Gain  Gain=-sim_.k_ang_vel  Multiplication=Matrix(K*u)
  Gain2 : Gain  Gain=-sim_.k_att  Multiplication=Matrix(K*u)
  Math Function{,1..5} (6 alike) : Math  Operator=transpose  SignedPower=on  SaturateOnIntegerOverflow=on
  Product{,1..17} (18 alike) : Product  Multiplication=Matrix(*)
  Scope1 : Scope
  Scope4 : Scope
  Sqrt : Sqrt  SaturateOnIntegerOverflow=on
  Sqrt1 : Sqrt  SaturateOnIntegerOverflow=on
  Sum : Sum  Inputs=|+-
  Sum1 : Sum  Inputs=|+-
  Sum2 : Sum  Inputs=|++
  Sum3 : Sum  Inputs=+-+-
  Sum4 : Sum  Inputs=+++
  Torque_in_body_frame : Outport  VectorParamsAs1DForOutWhenUnconnected=off
  wires:
  R_d/1 -> [R_d]
  omega_d/1 -> [omega_d]
  omega_d_dot/1 -> [omega_d_dot]
  [R_d] -> Math Function/1
  Math Function/1 -> Product/1
  R/1 -> [R]
  omega/1 -> [omega]
  [R] -> Product/2
  Product/1 -> [C]
  [C] -> Math Function1/1
  Math Function1/1 -> Product1/1
  [omega] -> Sum1/1
  Product1/1 -> Sum1/2
  [omega_d] -> Product1/2
  Sum2/1 -> [tau_d]
  Gain/1 -> Sum2/1
  [Omega_tide] -> Gain/1
  [tau_d] -> Sum3/1
  [C] -> Product4/1
  Constant/1 -> Cross Matrix/1(A), Product4/2
  Cross Matrix/1(AX) -> Product5/1
  Product4/1 -> Product5/2
  [C] -> Product6/1
  Constant2/1 -> Cross Matrix1/1(A), Product6/2
  Cross Matrix1/1(AX) -> Product7/1
  Product6/1 -> Product7/2
  Product7/1 -> Sum4/2
  [C] -> Product8/1
  Constant1/1 -> Cross Matrix2/1(A), Product8/2
  Cross Matrix2/1(AX) -> Product9/1
  Product8/1 -> Product9/2
  Product9/1 -> Sum4/3
  Product5/1 -> Sum4/1
  Gain2/1 -> Sum2/2
  Sum3/1 -> Torque_in_body_frame/1
  Constant3/1 -> Product2/1
  Sum/1 -> Product2/2
  [Omega_tide] -> Cross Matrix3/1(A)
  [C] -> Math Function2/1
  Cross Matrix3/1(AX) -> Product3/1
  Math Function2/1 -> Product3/2
  Product3/1 -> Product10/1
  [omega_d] -> Product10/2
  Product10/1 -> Sum/1
  [C] -> Math Function3/1
  Math Function3/1 -> Product11/1
  [omega_d_dot] -> Product11/2
  Product11/1 -> Sum/2
  Product2/1 -> Sum3/4
  Product13/1 -> Sum3/3
  Product12/1 -> Product13/1
  [omega] -> Product13/2
  [omega] -> Cross Matrix5/1(A)
  Cross Matrix5/1(AX) -> Product12/1
  Constant5/1 -> Product12/2
  Product14/1 -> Product15/1
  [Omega_tide] -> Product15/2
  [Omega_tide] -> Cross Matrix4/1(A)
  Cross Matrix4/1(AX) -> Product14/1
  Constant6/1 -> Product14/2
  Product15/1 -> Sum3/2
  Sum4/1 -> Product16/2, Math Function4/1, Gain2/1
  Math Function4/1 -> Product16/1
  Product16/1 -> Sqrt/1
  Sqrt/1 -> Scope1/1
  Sum1/1 -> Math Function5/1, Product17/2, [Omega_tide]
  Math Function5/1 -> Product17/1
  Product17/1 -> Sqrt1/1
  Sqrt1/1 -> Scope4/1

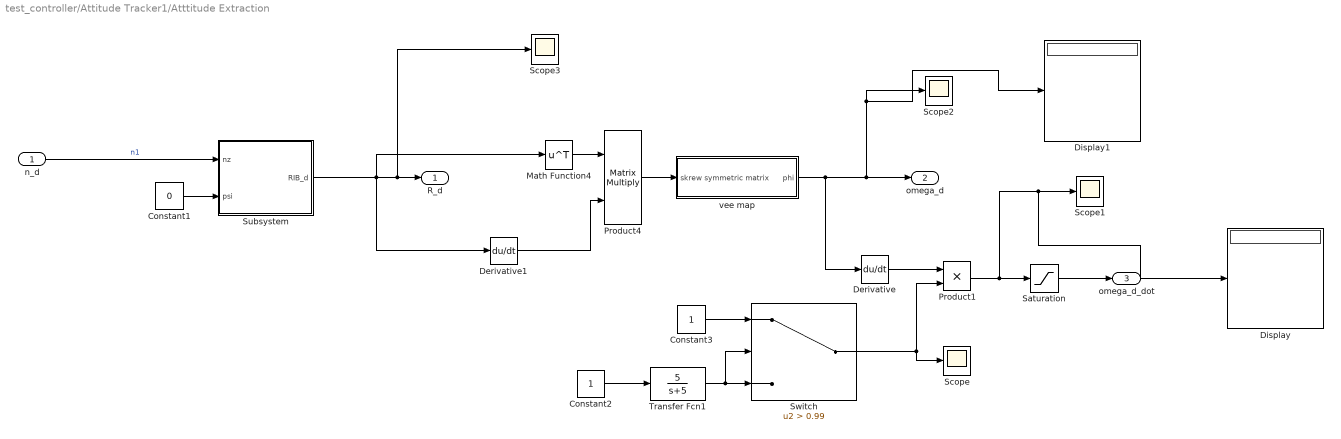
== system test_controller/Attitude Tracker1/Atttitude Extraction ==
  n_d : Inport
  Constant1 : Constant  Value=0
  Constant2 : Constant
  Constant3 : Constant
  Derivative : Derivative
  Derivative1 : Derivative
  Display : Display
  Display1 : Display
  Math Function4 : Math  Operator=transpose  SignedPower=on  SaturateOnIntegerOverflow=on
  Product1 : Product
  Product4 : Product  Multiplication=Matrix(*)
  Saturation : Saturate  UpperLimit=10  LowerLimit=-10
  Scope{,1..3} (4 alike) : Scope
  Subsystem : Subsystem
  Switch : Switch  Criteria=u2 > Threshold  Threshold=0.99  ZeroCross=off
  Transfer Fcn1 : TransferFcn  Numerator=[5]  Denominator=[1 5]
  vee map : Subsystem
  R_d : Outport  VectorParamsAs1DForOutWhenUnconnected=off
  omega_d : Outport  Port=2  VectorParamsAs1DForOutWhenUnconnected=off
  omega_d_dot : Outport  Port=3  VectorParamsAs1DForOutWhenUnconnected=off
  wires:
  Math Function4/1 -> Product4/1
  Derivative1/1 -> Product4/2
  Product4/1 -> vee map/1(skrew symmetric matrix)
  vee map/1(phi) -> Derivative/1, Display1/1, Scope2/1, omega_d/1
  n_d/1 -> Subsystem/1(nz)  "n1"
  Constant1/1 -> Subsystem/2(psi)
  Subsystem/1(RIB_d) -> Derivative1/1, Math Function4/1, Scope3/1, R_d/1
  Constant2/1 -> Transfer Fcn1/1
  Derivative/1 -> Product1/1
  Product1/1 -> Display/1, Scope1/1, Saturation/1
  Switch/1 -> Scope/1, Product1/2
  Constant3/1 -> Switch/1
  Transfer Fcn1/1 -> Switch/2, Switch/3
  Saturation/1 -> omega_d_dot/1

== system test_controller/B_hat & B_hat_dot1/Z ==
  y : Inport
  Constant : Constant  Value=params.derived.cable_len_sq  VectorParams1D=off
  Divide : Product  Inputs=*/
  Dot Product : DotProduct  InputSameDT=on  OutDataTypeStr=Inherit: Inherit via internal rule
  Dot Product1 : DotProduct  InputSameDT=on  OutDataTypeStr=Inherit: Inherit via internal rule
  Matrix Concatenate : Concatenate  ConcatenateDimension=2
  Sqrt : Sqrt  SaturateOnIntegerOverflow=on
  Sum : Sum  Inputs=|-+
  Transpose2 : Math  Operator=transpose  SignedPower=on  SaturateOnIntegerOverflow=on
  Z2 : Outport  VectorParamsAs1DForOutWhenUnconnected=off
  Z3/2 : Outport  Port=2  VectorParamsAs1DForOutWhenUnconnected=off
  y_T/Z : Outport  Port=3  VectorParamsAs1DForOutWhenUnconnected=off
  pld_rel_pos_full : Outport  Port=4  VectorParamsAs1DForOutWhenUnconnected=off
  wires:
  y/1 -> Divide/1, Matrix Concatenate/1, Dot Product/2, Dot Product/1
  Constant/1 -> Sum/2
  Dot Product/1 -> Sum/1
  Sum/1 -> Sqrt/1, Z2/1, Dot Product1/2
  Sqrt/1 -> Dot Product1/1, Divide/2, Matrix Concatenate/2
  Dot Product1/1 -> Z3/2/1
  Divide/1 -> Transpose2/1
  Transpose2/1 -> y_T/Z/1
  Matrix Concatenate/1 -> pld_rel_pos_full/1

== system test_controller/Guidance Law 1/normalize ==
  In1 : Inport
  Dot Product1 : DotProduct  InputSameDT=on  OutDataTypeStr=Inherit: Inherit via internal rule
  Product : Product
  Reciprocal Sqrt : Sqrt  Operator=rSqrt  SaturateOnIntegerOverflow=on
  Out1 : Outport
  wires:
  Dot Product1/1 -> Reciprocal Sqrt/1
  Reciprocal Sqrt/1 -> Product/2
  In1/1 -> Product/1, Dot Product1/2, Dot Product1/1
  Product/1 -> Out1/1

== system test_controller/Guidance Law 1/path_difference_sq ==
  p1 : Inport
  p2 : Inport  Port=2
  Dot Product : DotProduct  InputSameDT=on  OutDataTypeStr=Inherit: Inherit via internal rule
  Sum : Sum  Inputs=|+-
  sq dist : Outport
  wires:
  p1/1 -> Sum/1
  Sum/1 -> Dot Product/2, Dot Product/1
  Dot Product/1 -> sq dist/1
  p2/1 -> Sum/2

== system test_controller/Guidance Law 1/path_difference_sq1 ==
  p1 : Inport
  p2 : Inport  Port=2
  Dot Product : DotProduct  InputSameDT=on  OutDataTypeStr=Inherit: Inherit via internal rule
  Sum : Sum  Inputs=|+-
  sq dist : Outport
  wires:
  p1/1 -> Sum/1
  Sum/1 -> Dot Product/2, Dot Product/1
  Dot Product/1 -> sq dist/1
  p2/1 -> Sum/2

== system test_controller/Wind Disturbances/Wind_Profile ==
  note: Constant wind profile is used
  x : Inport
  Constant1 : Constant  Value=sim_.W_p
  Constant2 : Constant  Value=sim_.W_q
  Terminator : Terminator
  W_p : Outport  VectorParamsAs1DForOutWhenUnconnected=off
  W_q : Outport  Port=2  VectorParamsAs1DForOutWhenUnconnected=off
  wires:
  x/1 -> Terminator/1
  Constant2/1 -> W_q/1
  Constant1/1 -> W_p/1

== system test_controller/Attitude Tracker1/Attitude Dynamics/Cross Matrix ==
  A : Inport
  Constant1 : Constant  Value=0  VectorParams1D=off
  Constant2 : Constant  Value=0  VectorParams1D=off
  Constant3 : Constant  Value=0  VectorParams1D=off
  Demux2 : Demux  Outputs=3
  Gain : Gain  Gain=-1
  Gain1 : Gain  Gain=-1
  Gain2 : Gain  Gain=-1
  Matrix Concatenate : Concatenate  NumInputs=3  Mode=Multidimensional array  ConcatenateDimension=2
  Matrix Concatenate1 : Concatenate  NumInputs=3  Mode=Multidimensional array
  Matrix Concatenate2 : Concatenate  NumInputs=3  Mode=Multidimensional array
  Matrix Concatenate3 : Concatenate  NumInputs=3  Mode=Multidimensional array
  AX : Outport  VectorParamsAs1DForOutWhenUnconnected=off
  wires:
  A/1 -> Demux2/1
  Demux2/1 -> Gain1/1, Matrix Concatenate2/3  "r1"
  Demux2/2 -> Gain2/1, Matrix Concatenate3/1  "r2"
  Matrix Concatenate/1 -> AX/1
  Demux2/3 -> Gain/1, Matrix Concatenate1/2  "r3"
  Matrix Concatenate1/1 -> Matrix Concatenate/1
  Matrix Concatenate2/1 -> Matrix Concatenate/2
  Constant2/1 -> Matrix Concatenate2/2
  Gain/1 -> Matrix Concatenate2/1
  Matrix Concatenate3/1 -> Matrix Concatenate/3
  Gain1/1 -> Matrix Concatenate3/2
  Constant3/1 -> Matrix Concatenate3/3
  Constant1/1 -> Matrix Concatenate1/1
  Gain2/1 -> Matrix Concatenate1/3

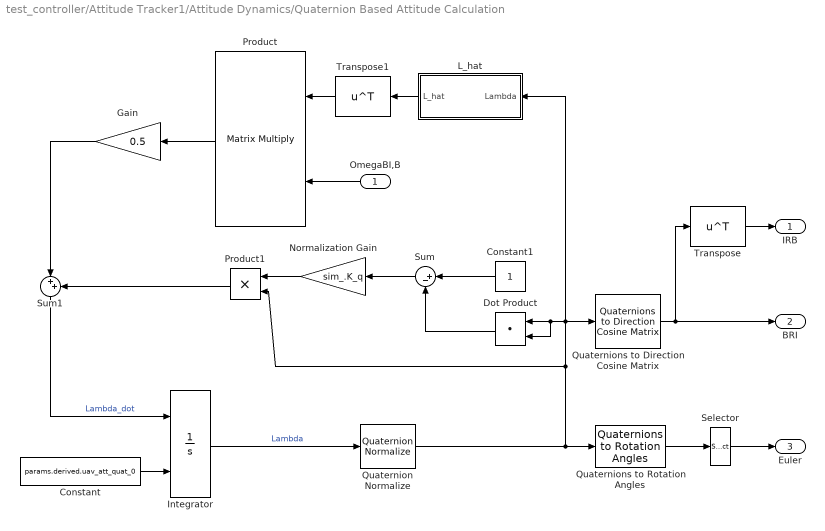
== system test_controller/Attitude Tracker1/Attitude Dynamics/Quaternion Based Attitude Calculation ==
  OmegaBI,B : Inport
  Constant : Constant  Value=params.derived.uav_att_quat_0
  Constant1 : Constant
  Dot Product : DotProduct  OutDataTypeStr=Inherit: Inherit via internal rule
  Gain : Gain  Gain=0.5
  Integrator : Integrator  InitialConditionSource=external
  L_hat : Subsystem
  Normalization Gain : Gain  Gain=sim_.K_q
  Product : Product  Multiplication=Matrix(*)  RndMeth=Zero
  Product1 : Product  RndMeth=Zero
  Quaternion Normalize : sharedutil/Quaternion Normalize  aMode=aMode
      settings: SourceProductBaseCode=AE,PW,MT,VE,VP
  Quaternions to Direction Cosine Matrix : sharedtransform/Quaternions to  Direction Cosine Matrix  aMode=aMode
      settings: SourceProductBaseCode=AE,PW,MT,VE,VP
  Quaternions to Rotation Angles : sharedtransform/Quaternions to Rotation Angles  rotationOrder=ZYX  aMode=aMode
      settings: SourceProductBaseCode=AE,PW,MT,VE,VP
  Selector : Selector  InputPortWidth=3  IndexOptions=Index vector (dialog)  Indices=[3 2 1]  OutputSizes=1
  Sum : Sum  Inputs=|+-  InputSameDT=on  SaturateOnIntegerOverflow=on  OutDataTypeStr=Inherit: Same as first input
  Sum1 : Sum  Inputs=|++
  Transpose : Math  Operator=transpose  SignedPower=on  SaturateOnIntegerOverflow=on
  Transpose1 : Math  Operator=transpose  SignedPower=on  SaturateOnIntegerOverflow=on
  IRB : Outport  VectorParamsAs1DForOutWhenUnconnected=off
  BRI : Outport  Port=2  VectorParamsAs1DForOutWhenUnconnected=off
  Euler : Outport  Port=3  VectorParamsAs1DForOutWhenUnconnected=off
  wires:
  Constant/1 -> Integrator/2
  Quaternions to Rotation Angles/1 -> Selector/1
  Selector/1 -> Euler/1
  Integrator/1 -> Quaternion Normalize/1  "Lambda"
  Sum1/1 -> Integrator/1  "Lambda_dot"
  Quaternions to Direction Cosine Matrix/1 -> BRI/1, Transpose/1
  Transpose/1 -> IRB/1
  Dot Product/1 -> Sum/2
  Constant1/1 -> Sum/1
  L_hat/1(L_hat) -> Transpose1/1
  Transpose1/1 -> Product/1
  OmegaBI,B/1 -> Product/2
  Sum/1 -> Normalization Gain/1
  Product/1 -> Gain/1
  Gain/1 -> Sum1/1
  Normalization Gain/1 -> Product1/1
  Product1/1 -> Sum1/2
  Quaternion Normalize/1 -> Quaternions to Rotation Angles/1, Quaternions to Direction Cosine Matrix/1, Dot Product/1, Dot Product/2, L_hat/1(Lambda), Product1/2

== system test_controller/Attitude Tracker1/Attitude Tracker/Cross Matrix ==
  A : Inport
  Constant1 : Constant  Value=0  VectorParams1D=off
  Constant2 : Constant  Value=0  VectorParams1D=off
  Constant3 : Constant  Value=0  VectorParams1D=off
  Demux2 : Demux  Outputs=3
  Gain : Gain  Gain=-1
  Gain1 : Gain  Gain=-1
  Gain2 : Gain  Gain=-1
  Matrix Concatenate : Concatenate  NumInputs=3  Mode=Multidimensional array  ConcatenateDimension=2
  Matrix Concatenate1 : Concatenate  NumInputs=3  Mode=Multidimensional array
  Matrix Concatenate2 : Concatenate  NumInputs=3  Mode=Multidimensional array
  Matrix Concatenate3 : Concatenate  NumInputs=3  Mode=Multidimensional array
  AX : Outport  VectorParamsAs1DForOutWhenUnconnected=off
  wires:
  A/1 -> Demux2/1
  Demux2/1 -> Gain1/1, Matrix Concatenate2/3  "r1"
  Demux2/2 -> Gain2/1, Matrix Concatenate3/1  "r2"
  Matrix Concatenate/1 -> AX/1
  Demux2/3 -> Gain/1, Matrix Concatenate1/2  "r3"
  Matrix Concatenate1/1 -> Matrix Concatenate/1
  Matrix Concatenate2/1 -> Matrix Concatenate/2
  Constant2/1 -> Matrix Concatenate2/2
  Gain/1 -> Matrix Concatenate2/1
  Matrix Concatenate3/1 -> Matrix Concatenate/3
  Gain1/1 -> Matrix Concatenate3/2
  Constant3/1 -> Matrix Concatenate3/3
  Constant1/1 -> Matrix Concatenate1/1
  Gain2/1 -> Matrix Concatenate1/3

== system test_controller/Attitude Tracker1/Attitude Tracker/Cross Matrix1 ==
  A : Inport
  Constant1 : Constant  Value=0  VectorParams1D=off
  Constant2 : Constant  Value=0  VectorParams1D=off
  Constant3 : Constant  Value=0  VectorParams1D=off
  Demux2 : Demux  Outputs=3
  Gain : Gain  Gain=-1
  Gain1 : Gain  Gain=-1
  Gain2 : Gain  Gain=-1
  Matrix Concatenate : Concatenate  NumInputs=3  Mode=Multidimensional array  ConcatenateDimension=2
  Matrix Concatenate1 : Concatenate  NumInputs=3  Mode=Multidimensional array
  Matrix Concatenate2 : Concatenate  NumInputs=3  Mode=Multidimensional array
  Matrix Concatenate3 : Concatenate  NumInputs=3  Mode=Multidimensional array
  AX : Outport  VectorParamsAs1DForOutWhenUnconnected=off
  wires:
  A/1 -> Demux2/1
  Demux2/1 -> Gain1/1, Matrix Concatenate2/3  "r1"
  Demux2/2 -> Gain2/1, Matrix Concatenate3/1  "r2"
  Matrix Concatenate/1 -> AX/1
  Demux2/3 -> Gain/1, Matrix Concatenate1/2  "r3"
  Matrix Concatenate1/1 -> Matrix Concatenate/1
  Matrix Concatenate2/1 -> Matrix Concatenate/2
  Constant2/1 -> Matrix Concatenate2/2
  Gain/1 -> Matrix Concatenate2/1
  Matrix Concatenate3/1 -> Matrix Concatenate/3
  Gain1/1 -> Matrix Concatenate3/2
  Constant3/1 -> Matrix Concatenate3/3
  Constant1/1 -> Matrix Concatenate1/1
  Gain2/1 -> Matrix Concatenate1/3

== system test_controller/Attitude Tracker1/Attitude Tracker/Cross Matrix2 ==
  A : Inport
  Constant1 : Constant  Value=0  VectorParams1D=off
  Constant2 : Constant  Value=0  VectorParams1D=off
  Constant3 : Constant  Value=0  VectorParams1D=off
  Demux2 : Demux  Outputs=3
  Gain : Gain  Gain=-1
  Gain1 : Gain  Gain=-1
  Gain2 : Gain  Gain=-1
  Matrix Concatenate : Concatenate  NumInputs=3  Mode=Multidimensional array  ConcatenateDimension=2
  Matrix Concatenate1 : Concatenate  NumInputs=3  Mode=Multidimensional array
  Matrix Concatenate2 : Concatenate  NumInputs=3  Mode=Multidimensional array
  Matrix Concatenate3 : Concatenate  NumInputs=3  Mode=Multidimensional array
  AX : Outport  VectorParamsAs1DForOutWhenUnconnected=off
  wires:
  A/1 -> Demux2/1
  Demux2/1 -> Gain1/1, Matrix Concatenate2/3  "r1"
  Demux2/2 -> Gain2/1, Matrix Concatenate3/1  "r2"
  Matrix Concatenate/1 -> AX/1
  Demux2/3 -> Gain/1, Matrix Concatenate1/2  "r3"
  Matrix Concatenate1/1 -> Matrix Concatenate/1
  Matrix Concatenate2/1 -> Matrix Concatenate/2
  Constant2/1 -> Matrix Concatenate2/2
  Gain/1 -> Matrix Concatenate2/1
  Matrix Concatenate3/1 -> Matrix Concatenate/3
  Gain1/1 -> Matrix Concatenate3/2
  Constant3/1 -> Matrix Concatenate3/3
  Constant1/1 -> Matrix Concatenate1/1
  Gain2/1 -> Matrix Concatenate1/3

== system test_controller/Attitude Tracker1/Attitude Tracker/Cross Matrix3 ==
  A : Inport
  Constant1 : Constant  Value=0  VectorParams1D=off
  Constant2 : Constant  Value=0  VectorParams1D=off
  Constant3 : Constant  Value=0  VectorParams1D=off
  Demux2 : Demux  Outputs=3
  Gain : Gain  Gain=-1
  Gain1 : Gain  Gain=-1
  Gain2 : Gain  Gain=-1
  Matrix Concatenate : Concatenate  NumInputs=3  Mode=Multidimensional array  ConcatenateDimension=2
  Matrix Concatenate1 : Concatenate  NumInputs=3  Mode=Multidimensional array
  Matrix Concatenate2 : Concatenate  NumInputs=3  Mode=Multidimensional array
  Matrix Concatenate3 : Concatenate  NumInputs=3  Mode=Multidimensional array
  AX : Outport  VectorParamsAs1DForOutWhenUnconnected=off
  wires:
  A/1 -> Demux2/1
  Demux2/1 -> Gain1/1, Matrix Concatenate2/3  "r1"
  Demux2/2 -> Gain2/1, Matrix Concatenate3/1  "r2"
  Matrix Concatenate/1 -> AX/1
  Demux2/3 -> Gain/1, Matrix Concatenate1/2  "r3"
  Matrix Concatenate1/1 -> Matrix Concatenate/1
  Matrix Concatenate2/1 -> Matrix Concatenate/2
  Constant2/1 -> Matrix Concatenate2/2
  Gain/1 -> Matrix Concatenate2/1
  Matrix Concatenate3/1 -> Matrix Concatenate/3
  Gain1/1 -> Matrix Concatenate3/2
  Constant3/1 -> Matrix Concatenate3/3
  Constant1/1 -> Matrix Concatenate1/1
  Gain2/1 -> Matrix Concatenate1/3

== system test_controller/Attitude Tracker1/Attitude Tracker/Cross Matrix4 ==
  A : Inport
  Constant1 : Constant  Value=0  VectorParams1D=off
  Constant2 : Constant  Value=0  VectorParams1D=off
  Constant3 : Constant  Value=0  VectorParams1D=off
  Demux2 : Demux  Outputs=3
  Gain : Gain  Gain=-1
  Gain1 : Gain  Gain=-1
  Gain2 : Gain  Gain=-1
  Matrix Concatenate : Concatenate  NumInputs=3  Mode=Multidimensional array  ConcatenateDimension=2
  Matrix Concatenate1 : Concatenate  NumInputs=3  Mode=Multidimensional array
  Matrix Concatenate2 : Concatenate  NumInputs=3  Mode=Multidimensional array
  Matrix Concatenate3 : Concatenate  NumInputs=3  Mode=Multidimensional array
  AX : Outport  VectorParamsAs1DForOutWhenUnconnected=off
  wires:
  A/1 -> Demux2/1
  Demux2/1 -> Gain1/1, Matrix Concatenate2/3  "r1"
  Demux2/2 -> Gain2/1, Matrix Concatenate3/1  "r2"
  Matrix Concatenate/1 -> AX/1
  Demux2/3 -> Gain/1, Matrix Concatenate1/2  "r3"
  Matrix Concatenate1/1 -> Matrix Concatenate/1
  Matrix Concatenate2/1 -> Matrix Concatenate/2
  Constant2/1 -> Matrix Concatenate2/2
  Gain/1 -> Matrix Concatenate2/1
  Matrix Concatenate3/1 -> Matrix Concatenate/3
  Gain1/1 -> Matrix Concatenate3/2
  Constant3/1 -> Matrix Concatenate3/3
  Constant1/1 -> Matrix Concatenate1/1
  Gain2/1 -> Matrix Concatenate1/3
